simulink model "digital_smps"  (R2022a)
settings: Solver=ode45  StartTime=0.0  StopTime=0.01  MaxStep=0.1e-6  RelTol=1e-3  EnableMultiTasking=on
settings Model: Creator=Rieri  LastModifiedBy=emman
settings SolverCC: AlgebraicLoopSolver=TrustRegion
settings DataIOCC: LimitDataPoints=on  SaveFormat=Array  SignalLoggingSaveFormat=ModelDataLogs  ReturnWorkspaceOutputs=off
settings DebuggingCC: SaveWithParameterizedLinksMsg=none  UnderspecifiedInitializationDetection=Classic  MergeDetectMultiDrivingBlocksExec=none  SignalResolutionControl=TryResolveAllWithWarning  MultiTaskDSMMsg=warning  MultiTaskCondExecSysMsg=none  UnconnectedInputMsg=warning  UnconnectedOutputMsg=warning  UnconnectedLineMsg=warning  SFMachineParentedDataDiag=warning
settings HardwareCC: TargetUnknown=on
settings ModelReferenceCC: PropagateSignalLabelsOutOfModel=off
settings RTWCC: DLArmComputeVersion=19.05
settings GRTTargetCC: CombineOutputUpdateFcns=off  GRTInterface=on

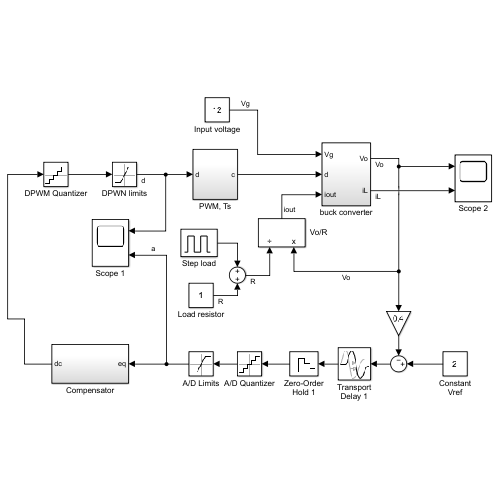
[thumbnail: Simulink's stored preview of the top-level diagram]
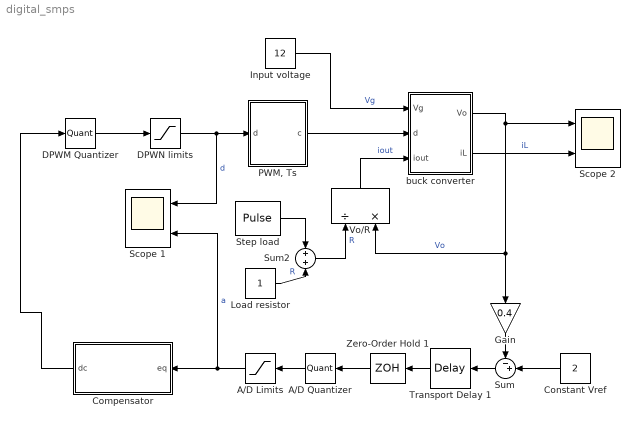
== system digital_smps ==
  A/D Limits : Saturate  UpperLimit=5  LowerLimit=-5
  A/D Quantizer : Quantizer  QuantizationInterval=1/(2^8)
  Compensator : Subsystem
  Constant Vref : Constant  Value=2
  DPWM Quantizer : Quantizer  QuantizationInterval=1/(2^8)
  DPWN limits : Saturate  UpperLimit=1  LowerLimit=-1
  Gain : Gain  Gain=0.4  SaturateOnIntegerOverflow=on
  Input voltage : Constant  Value=12
  Load resistor : Constant
  "PWM, Ts" : Subsystem
  Scope 1 : Scope  NumInputPorts=2
  Scope 2 : Scope  NumInputPorts=2
  Step load : DiscretePulseGenerator  PulseType=Time based  Amplitude=10  Period=0.02  PulseWidth=50
  Sum : Sum  Inputs=-+|  SaturateOnIntegerOverflow=on
  Sum2 : Sum  Inputs=+|+  SaturateOnIntegerOverflow=on
  Transport Delay 1 : TransportDelay  DelayTime=0.0001
  Vo/R : Product  Inputs=/*  SaturateOnIntegerOverflow=on
  Zero-Order Hold 1 : ZeroOrderHold  SampleTime=1/220000
  buck converter : Subsystem
  wires:
  Input voltage/1 -> buck converter/1(Vg)  "Vg"
  buck converter/1(Vo) -> Vo/R/2, Gain/1, Scope 2/1  "Vo"
  Vo/R/1 -> buck converter/3(iout)  "iout"
  Gain/1 -> Sum/1
  Constant Vref/1 -> Sum/2
  Load resistor/1 -> Sum2/2  "R"
  Sum2/1 -> Vo/R/1  "R"
  "PWM, Ts"/1(c) -> buck converter/2(d)
  buck converter/2(iL) -> Scope 2/2  "iL"
  Step load/1 -> Sum2/1
  Zero-Order Hold 1/1 -> A/D Quantizer/1
  A/D Quantizer/1 -> A/D Limits/1
  DPWM Quantizer/1 -> DPWN limits/1
  A/D Limits/1 -> Scope 1/2, Compensator/1(eq)  "a"
  Compensator/1(dc) -> DPWM Quantizer/1
  DPWN limits/1 -> Scope 1/1, "PWM, Ts"/1(d)  "d"
  Transport Delay 1/1 -> Zero-Order Hold 1/1
  Sum/1 -> Transport Delay 1/1

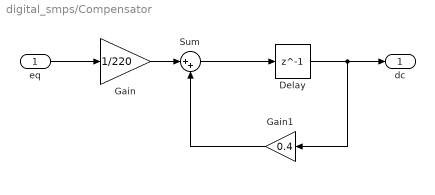
== system digital_smps/Compensator ==
  eq : Inport
  Delay : Delay  DelayLength=1  InitialCondition=0
  Gain : Gain  Gain=1/220
  Gain1 : Gain  Gain=0.4
  Sum : Sum  Inputs=|++
  dc : Outport
  wires:
  eq/1 -> Gain/1
  Gain/1 -> Sum/1
  Sum/1 -> Delay/1
  Delay/1 -> Gain1/1, dc/1
  Gain1/1 -> Sum/2

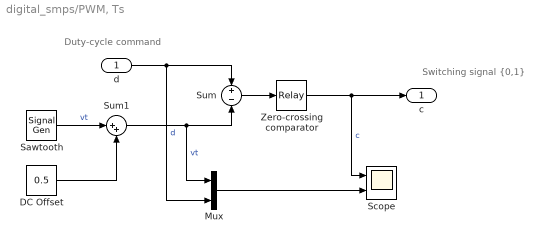
== system digital_smps/PWM, Ts ==
  note: Switching signal {0,1}
  note: Duty-cycle
      | command
  d : Inport
  DC Offset : Constant  Value=0.5
  Mux : Mux  Inputs=2
  Sawtooth : SignalGenerator  WaveForm=sawtooth  Amplitude=-0.5  Frequency=100000
  Scope : Scope  NumInputPorts=2
  Sum : Sum  Inputs=+|-  SaturateOnIntegerOverflow=on
  Sum1 : Sum  Inputs=|++
  Zero-crossing comparator : Relay
  c : Outport
  wires:
  DC Offset/1 -> Sum1/2
  Sum/1 -> Zero-crossing comparator/1
  Mux/1 -> Scope/2
  Zero-crossing comparator/1 -> c/1, Scope/1  "c"
  Sawtooth/1 -> Sum1/1  "vt"
  Sum1/1 -> Mux/1, Sum/2  "vt"
  d/1 -> Mux/2, Sum/1  "d"

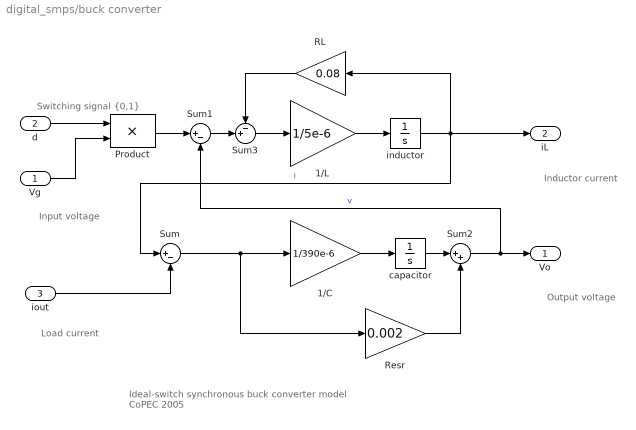
== system digital_smps/buck converter ==
  note: Load current
  note: Input voltage
  note: Inductor current
  note: Output voltage
  note: Switching signal {0,1}
  note: Ideal-switch synchronous buck converter model
      | CoPEC 2005
  Vg : Inport
  d : Inport  Port=2
  iout : Inport  Port=3
  1/C : Gain  Gain=1/390e-6  SaturateOnIntegerOverflow=on
  1/L : Gain  Gain=1/5e-6  SaturateOnIntegerOverflow=on
  Product : Product  SaturateOnIntegerOverflow=on
  RL : Gain  Gain=0.08  SaturateOnIntegerOverflow=on
  Resr : Gain  Gain=0.002  SaturateOnIntegerOverflow=on
  Sum : Sum  Inputs=|+-  SaturateOnIntegerOverflow=on
  Sum1 : Sum  Inputs=|+-  SaturateOnIntegerOverflow=on
  Sum2 : Sum  Inputs=|++  SaturateOnIntegerOverflow=on
  Sum3 : Sum  Inputs=-+|  SaturateOnIntegerOverflow=on
  capacitor : Integrator
  inductor : Integrator
  Vo : Outport
  iL : Outport  Port=2
  wires:
  iout/1 -> Sum/2
  d/1 -> Product/1
  Resr/1 -> Sum2/2
  capacitor/1 -> Sum2/1
  Sum3/1 -> 1/L/1
  RL/1 -> Sum3/1
  Sum1/1 -> Sum3/2
  Sum2/1 -> Sum1/2, Vo/1  "v"
  Product/1 -> Sum1/1
  inductor/1 -> Sum/1, RL/1, iL/1  "i"
  1/L/1 -> inductor/1
  Sum/1 -> 1/C/1, Resr/1
  1/C/1 -> capacitor/1
  Vg/1 -> Product/2
